simulink model "psbxfosaturable"  (Simulink 6.0)
settings: Solver=ode15s  SolverMode=SingleTasking  StartTime=0.0  StopTime=0.5  RelTol=1e-3  AbsTol=1e-2
libraries: powerlib2 x10
settings Model: Creator=patrice  LastModifiedBy=batserve  ExtModeTrigMode=oneshot  ExtModeArmWhenConnect=off  ExtModeAutoUpdateStatusClock=off
settings DataIOCC: LimitDataPoints=off  SignalLoggingName=sigsOut
settings OptimizationCC: BlockReduction=off  BooleanDataType=off
settings DebuggingCC: SolverPrmCheckMsg=none
settings HardwareCC: TargetUnknown=on
settings RTWCC: TemplateMakefile=grt_unix.tmf

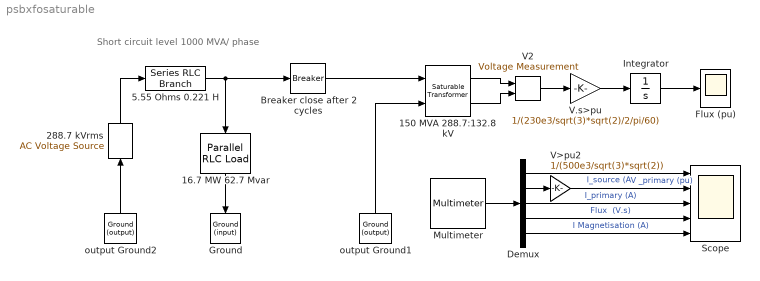
== system psbxfosaturable ==
  note: Short circuit level
      | 1000 MVA/ phase
  150 MVA 288.7:132.8 kV : powerlib2/Elements/Saturable Transformer  Tag=PoWeRsYsTeMbLoCk  a=[ 150e6 60 ]  b=[ 500e3/sqrt(3) 0.002 0.08 ]  c=[ 230e3/sqrt(3) 0.002 0.08]  w3check=off  d=[ 230e3/sqrt(3) 0.002 0.08]  e="[0 0;  0.0 1.2; 1.0  1.52]"  f=[500 0.8]  H=off  matfile='hysteresis_SI'  Initialslope=+1  mesure=All measurements (V I Flux)  PSBOutputType=1111
  16.7 MW 62.7 Mvar : powerlib2/Elements/Parallel RLC Load  Tag=PoWeRsYsTeMbLoCk  Orientation=down  a=500e3/sqrt(3)  b=60  c=16.7e6  d=0  e=62.7e6  mesure=None  PSBOutputType=1
  288.7 kVrms : powerlib2/Electrical Sources/AC Voltage Source  Tag=PoWeRsYsTeMbLoCk  Orientation=up  A=500e3/sqrt(3)*sqrt(2)  P=0  F=60  stime=0  mesure=None  PSBOutputType=1
  "5.55 Ohms 0.221 H " : powerlib2/Elements/Series RLC Branch  Tag=PoWeRsYsTeMbLoCk  a=5.55  b=0.221  c=inf  mesure=Branch current  PSBOutputType=1
  Breaker close after 2 cycles : powerlib2/Elements/Breaker  Tag=PoWeRsYsTeMbLoCk  a=0.01  c=0  rs=100e6  cs=inf  times=[ 2/60 ]  Ts=0  comext=off  mesure=None  PSBOutputType=1
  Demux : Demux  Outputs=5
  Flux (pu) : Scope
      settings: DeleteFcn=simscope BlockIsBeingDestroyed  PostSaveFcn=simscope Save  TickLabels=on  TimeRange=0.5  YMin=-0.25  YMax=2.25  DataFormat=Array
  Ground : powerlib2/Connectors/Ground (input)  Tag=PoWeRsYsTeMbLoCk  Orientation=down
  Integrator : Integrator  InitialCondition=0.8
  Multimeter : powerlib2/Measurements/Multimeter  Tag=PoWeRsYsTeMmEaSuReMeNt  PhasorSimulation=off  OutputType=Magnitude  sel=[3 1 4 8 6]  L=8  Gain=[1 1 1 1 1]  yselected=[2,8.0017089843750000e+000;3,5.0018310546875000e+000;6,5.0018310546875000e+000;16,5.0018310546875000e+000;9,5.0018310546875000e+000]  PSBOutputType=1  PSBequivalent=0  AxesSetting=[0,0.1,-100,100]  Display=0  SavedBlockNames=-11
  Scope : Scope  NumInputPorts=5
      settings: DeleteFcn=simscope BlockIsBeingDestroyed  PostSaveFcn=simscope Save  TimeRange=0.5  YMin=-500~-1.5~-500~0~-500  YMax=2500~1.5~2500~2500~2500  SaveName=R
  V.s>pu : Gain  Gain=1/(230e3/sqrt(3)*sqrt(2)/2/pi/60)  SaturateOnIntegerOverflow=on
  V2 : powerlib2/Measurements/Voltage Measurement  Tag=PoWeRsYsTeMmEaSuReMeNt  PhasorSimulation=off  OutputType=Magnitude  PSBOutputType=0  PSBequivalent=0
  V>pu2 : Gain  Gain=1/(500e3/sqrt(3)*sqrt(2))  SaturateOnIntegerOverflow=on
  output Ground1 : powerlib2/Connectors/Ground (output)  Tag=PoWeRsYsTeMbLoCk  Orientation=up  PSBOutputType=1
  output Ground2 : powerlib2/Connectors/Ground (output)  Tag=PoWeRsYsTeMbLoCk  Orientation=up  PSBOutputType=1
  wires:
  288.7 kVrms/1 -> "5.55 Ohms 0.221 H "/1
  output Ground2/1 -> 288.7 kVrms/1
  "5.55 Ohms 0.221 H "/1 -> 16.7 MW 62.7 Mvar/1, Breaker close after 2 cycles/1
  16.7 MW 62.7 Mvar/1 -> Ground/1
  output Ground1/1 -> 150 MVA 288.7:132.8 kV/2
  Breaker close after 2 cycles/1 -> 150 MVA 288.7:132.8 kV/1
  150 MVA 288.7:132.8 kV/1 -> V2/1
  150 MVA 288.7:132.8 kV/2 -> V2/2
  V2/1 -> V.s>pu/1
  Integrator/1 -> Flux (pu)/1
  V.s>pu/1 -> Integrator/1
  Multimeter/1 -> Demux/1
  Demux/1 -> Scope/1  "I_source (A)"
  Demux/3 -> Scope/3  "I_primary (A)"
  Demux/4 -> Scope/4  "Flux  (V.s)"
  Demux/2 -> V>pu2/1
  V>pu2/1 -> Scope/2  "V _primary (pu)"
  Demux/5 -> Scope/5  "I Magnetisation (A)"
